simulink model "walkingRobotCapture"  (R2020a)
settings: Solver=ode15s  StartTime=0.0  StopTime=inf  EnableMultiTasking=on
PreLoadFcn:
  | % run script to load up the parameters
  | robotParameters
values from neighbouring files (symbols this model uses):
  foot_x = 0.17    [robotParameters.m]
  foot_y = 0.17    [robotParameters.m]
  foot_z = 0.02    [robotParameters.m]
  init_angs_L = zeros(6,1)    [robotParameters.m]
  init_angs_R = zeros(6,1)    [robotParameters.m]
  leg_width = 0.08    [robotParameters.m]
  lower_leg_length = 0.38    [robotParameters.m]
  plane_x = 3    [robotParameters.m]    (also in startupWalkingRobot.m = 30)
  plane_y = 50    [robotParameters.m]
  plane_z = height_plane    (= 0.025)    [robotParameters.m]
  s = Rp(:,2)    [invKinBody2Foot.m]
  torso_height = 0.35    [robotParameters.m]
  torso_length = 0.20    (= 0.2)    [robotParameters.m]
  torso_offset_height = 0    [robotParameters.m]
  torso_offset_length = 0    [robotParameters.m]
  torso_width = 0.24    [robotParameters.m]
  Ts = 0.005    [startupWalkingRobot.m]
  upper_leg_length = 0.40    (= 0.4)    [robotParameters.m]
  X = mat(1,4)    [Transform.m]
  Y = mat(2,4)    [Transform.m]
  Z = mat(3,4)    [Transform.m]
libraries: sm_lib x57, walkingRobotUtils x17, nesl_utility x4, simulink x1
(part 2 of 3)

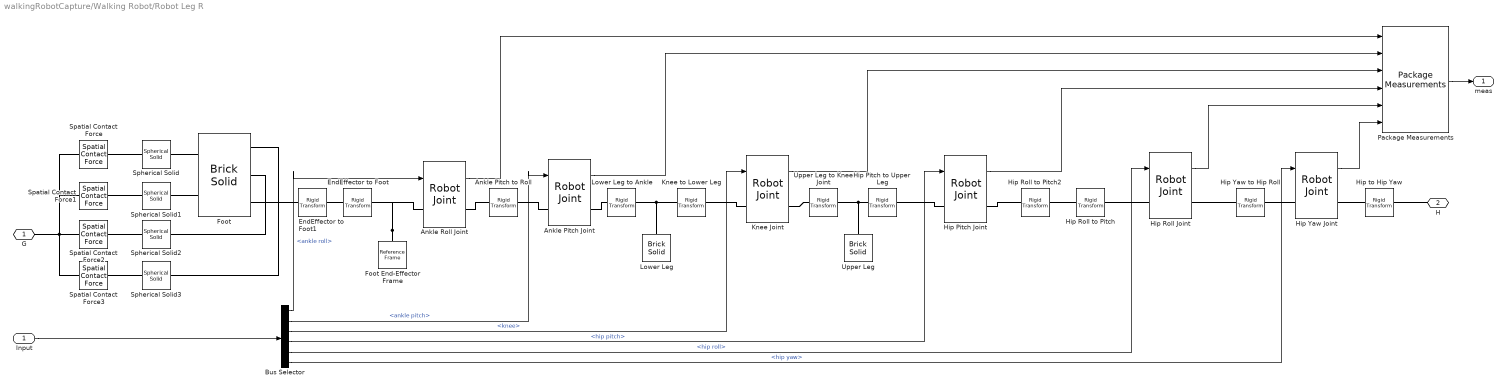
== system walkingRobotCapture/Walking Robot/Robot Leg R ==
  Input : Inport
  Ankle Pitch Joint : walkingRobotUtils/Robot Joint  jointDamping=joint_damping  initAngle=init_angs_R(5)  upperLimit=pi/2  lowerLimit=-pi/2  limitK=1000  limitD=100
  Ankle Pitch to Roll : sm_lib/Frames and Transforms/Rigid Transform  TranslationMethod=None  TranslationStandardOffset=0  TranslationLengthUnit=cm  TranslationStandardAxis=+Z  TranslationCartesianOffset=[0 0 upper_leg_length/2]  TranslationROffset=0  TranslationROffsetUnits=m  TranslationZOffset=0  TranslationZOffsetUnits=m  TranslationThetaOffset=0  TranslationThetaOffsetUnits=deg  RotationMethod=StandardAxis  RotationAngleUnits=deg  RotationStandardAxis=+X  RotationAngle=90  RotationArbitraryAxis=[0 0 1]  FollAlignAxisA=+X  BaseAlignAxisA=+Y  FollAlignAxisB=+Y  BaseAlignAxisB=+Z  RotationSequenceAxes=FollowerAxes  RotationSequence=XYX  RotationSequenceAngles=[0 0 0]  RotationSequenceAnglesUnits=deg  RotationMatrix=[1 0 0; 0 1 0; 0 0 1]
  Ankle Roll Joint : walkingRobotUtils/Robot Joint  jointDamping=joint_damping  initAngle=init_angs_R(6)  upperLimit=pi/2  lowerLimit=-pi/2  limitK=1000  limitD=100
  Bus Selector : BusSelector  OutputSignals=ankle roll,ankle pitch,knee,hip pitch,hip roll,hip yaw
  EndEffector to Foot : sm_lib/Frames and Transforms/Rigid Transform  TranslationMethod=None  TranslationStandardOffset=0  TranslationLengthUnit=cm  TranslationStandardAxis=+Z  TranslationCartesianOffset=[0 0 upper_leg_length/2]  TranslationROffset=0  TranslationROffsetUnits=m  TranslationZOffset=0  TranslationZOffsetUnits=m  TranslationThetaOffset=0  TranslationThetaOffsetUnits=deg  RotationMethod=StandardAxis  RotationAngleUnits=deg  RotationStandardAxis=+Z  RotationAngle=-90  RotationArbitraryAxis=[0 0 1]  FollAlignAxisA=+X  BaseAlignAxisA=+Y  FollAlignAxisB=+Y  BaseAlignAxisB=+Z  RotationSequenceAxes=FollowerAxes  RotationSequence=XYX  RotationSequenceAngles=[0 0 0]  RotationSequenceAnglesUnits=deg  RotationMatrix=[1 0 0; 0 1 0; 0 0 1]
  EndEffector to Foot1 : sm_lib/Frames and Transforms/Rigid Transform  TranslationMethod=None  TranslationStandardOffset=0  TranslationLengthUnit=cm  TranslationStandardAxis=+Z  TranslationCartesianOffset=[0 0 upper_leg_length/2]  TranslationROffset=0  TranslationROffsetUnits=m  TranslationZOffset=0  TranslationZOffsetUnits=m  TranslationThetaOffset=0  TranslationThetaOffsetUnits=deg  RotationMethod=StandardAxis  RotationAngleUnits=deg  RotationStandardAxis=+X  RotationAngle=180  RotationArbitraryAxis=[0 0 1]  FollAlignAxisA=+X  BaseAlignAxisA=+Y  FollAlignAxisB=+Y  BaseAlignAxisB=+Z  RotationSequenceAxes=FollowerAxes  RotationSequence=XYX  RotationSequenceAngles=[0 0 0]  RotationSequenceAnglesUnits=deg  RotationMatrix=[1 0 0; 0 1 0; 0 0 1]
  Foot : sm_lib/Body Elements/Brick Solid  GraphicAmbientColor=[0.15 0.15 0.15 1.0]  BasedOnType=Density  BrickDimensions=[foot_x foot_y foot_z]  BrickDimensionUnits=m  CenterOfMass=[0 0 0]  CenterOfMassUnits=m  GraphicDiffuseColor=[0.5 0.5 0.5]  Density=200  DensityUnits=kg/(m^3)  DoExposeReferenceFrame=off  GraphicEmissiveColor=[0.0 0.0 0.0 1.0]  ExportEntireGeometry=off  SerializedFrames=<Frames><Frame><Id>Frame1</Id><Value><Name>F1</Name><Origin><Source>GeometricFeature</Source><FeatureName>+x -y curve</FeatureName></Origin><PrimaryAxis><DefinedDirection>+Z</DefinedDirection><Source>ReferenceFrame</Source><SourceDirection>+Z</SourceDirection><FeatureName></FeatureName></PrimaryAxis><SecondaryAxis><DefinedDirection>+X</DefinedDirection><Source>ReferenceFrame</Source><SourceDirection>+X</SourceDirection><FeatureName></FeatureName></SecondaryAxis></Value></Frame><Frame><Id>Frame2</Id><Value><Name>F2</Name><Origin><Source>GeometricFeature</Source><FeatureName>+x +y curve</FeatureName></Origin><PrimaryAxis><DefinedDirection>+Z</DefinedDirection><Source>ReferenceFrame</Source><SourceDirection>+Z</SourceDirection><FeatureName></FeatureName></PrimaryAxis><SecondaryAxis><DefinedDirection>+X</DefinedDirection><Source>ReferenceFrame</Source><SourceDirection>+X</SourceDirection><FeatureName></FeatureName></SecondaryAxis></Value></Frame><Frame><Id>Frame3</Id><Value><Name>F3</Name><Origin><Source>GeometricFeature</Source><FeatureName>-x -y curve</FeatureName></Origin><PrimaryAxis><DefinedDirection>+Z</DefinedDirection><Source>ReferenceFrame</Source><SourceDirection>+Z</SourceDirection><FeatureName></FeatureName></PrimaryAxis><SecondaryAxis><DefinedDirection>+X</DefinedDirection><Source>ReferenceFrame</Source><SourceDirection>+X</SourceDirection><FeatureName></FeatureName></SecondaryAxis></Value></Frame><Frame><Id>Frame4</Id><Value><Name>F4</Name><Origin><Source>GeometricFeature</Source><FeatureName>-x +y curve</FeatureName></Origin><PrimaryAxis><DefinedDirection>+Z</DefinedDirection><Source>ReferenceFrame</Source><SourceDirection>+Z</SourceDirection><FeatureName></FeatureName></PrimaryAxis><SecondaryAxis><DefinedDirection>+X</DefinedDirection><Source>ReferenceFrame</Source><SourceDirection>+X</SourceDirection><FeatureName></FeatureName></SecondaryAxis></Value></Frame><Frame><Id>Frame5</Id><Value><Name>A</Name><Origin><Source>GeometricFeature</Source><FeatureName>+z surface</FeatureName></Origin><PrimaryAxis><DefinedDirection>+Z</DefinedDirection><Source>ReferenceFrame</Source><SourceDirection>-Y</SourceDirection><FeatureName></FeatureName></PrimaryAxis><SecondaryAxis><DefinedDirection>+X</DefinedDirection><Source>ReferenceFrame</Source><SourceDirection>+X</SourceDirection><FeatureName></FeatureName></SecondaryAxis></Value></Frame></Frames>  MarkerShape=Sphere  MarkerSize=10  GraphicType=FromGeometry  InertiaType=CalculateFromGeometry  Mass=1  MassUnits=kg  MomentsOfInertia=[1 1 1]  MomentsOfInertiaUnits=kg*m^2  GraphicOpacity=1.0  ProductsOfInertia=[0 0 0]  ProductsOfInertiaUnits=kg*m^2  GraphicShininess=75  GraphicSpecularColor=[0.5 0.5 0.5 1.0]  GraphicVisPropType=SimpleVisualProperties
  Foot End-Effector Frame : sm_lib/Frames and Transforms/Reference Frame
  Hip Pitch Joint : walkingRobotUtils/Robot Joint  jointDamping=joint_damping  initAngle=init_angs_R(3)  upperLimit=pi/2  lowerLimit=-pi/2  limitK=1000  limitD=100
  Hip Pitch to Upper Leg : sm_lib/Frames and Transforms/Rigid Transform  TranslationMethod=StandardAxis  TranslationStandardOffset=upper_leg_length/2  TranslationLengthUnit=m  TranslationStandardAxis=+X  TranslationCartesianOffset=[upper_leg_length/2 0 0]  TranslationROffset=0  TranslationROffsetUnits=m  TranslationZOffset=0  TranslationZOffsetUnits=m  TranslationThetaOffset=0  TranslationThetaOffsetUnits=deg  RotationMethod=StandardAxis  RotationAngleUnits=deg  RotationStandardAxis=+Y  RotationAngle=90  RotationArbitraryAxis=[0 0 1]  FollAlignAxisA=+X  BaseAlignAxisA=+Y  FollAlignAxisB=+Y  BaseAlignAxisB=+Z  RotationSequenceAxes=FollowerAxes  RotationSequence=XYX  RotationSequenceAngles=[0 0 0]  RotationSequenceAnglesUnits=deg  RotationMatrix=[1 0 0; 0 1 0; 0 0 1]
  Hip Roll Joint : walkingRobotUtils/Robot Joint  jointDamping=joint_damping  initAngle=init_angs_R(2)  upperLimit=pi/2  lowerLimit=-pi/2  limitK=1000  limitD=100
  Hip Roll to Pitch : sm_lib/Frames and Transforms/Rigid Transform  TranslationMethod=None  TranslationStandardOffset=0  TranslationLengthUnit=cm  TranslationStandardAxis=+Z  TranslationCartesianOffset=[0 0 upper_leg_length/2]  TranslationROffset=0  TranslationROffsetUnits=m  TranslationZOffset=0  TranslationZOffsetUnits=m  TranslationThetaOffset=0  TranslationThetaOffsetUnits=deg  RotationMethod=StandardAxis  RotationAngleUnits=deg  RotationStandardAxis=+Z  RotationAngle=-90  RotationArbitraryAxis=[0 0 1]  FollAlignAxisA=+X  BaseAlignAxisA=+Y  FollAlignAxisB=+Y  BaseAlignAxisB=+Z  RotationSequenceAxes=FollowerAxes  RotationSequence=XYX  RotationSequenceAngles=[0 0 0]  RotationSequenceAnglesUnits=deg  RotationMatrix=[1 0 0; 0 1 0; 0 0 1]
  Hip Roll to Pitch2 : sm_lib/Frames and Transforms/Rigid Transform  TranslationMethod=None  TranslationStandardOffset=0  TranslationLengthUnit=cm  TranslationStandardAxis=+Z  TranslationCartesianOffset=[0 0 upper_leg_length/2]  TranslationROffset=0  TranslationROffsetUnits=m  TranslationZOffset=0  TranslationZOffsetUnits=m  TranslationThetaOffset=0  TranslationThetaOffsetUnits=deg  RotationMethod=StandardAxis  RotationAngleUnits=deg  RotationStandardAxis=+X  RotationAngle=-90  RotationArbitraryAxis=[0 0 1]  FollAlignAxisA=+X  BaseAlignAxisA=+Y  FollAlignAxisB=+Y  BaseAlignAxisB=+Z  RotationSequenceAxes=FollowerAxes  RotationSequence=XYX  RotationSequenceAngles=[0 0 0]  RotationSequenceAnglesUnits=deg  RotationMatrix=[1 0 0; 0 1 0; 0 0 1]
  Hip Yaw Joint : walkingRobotUtils/Robot Joint  jointDamping=joint_damping  initAngle=init_angs_R(1)  upperLimit=pi/2  lowerLimit=-pi/2  limitK=1000  limitD=100
  Hip Yaw to Hip Roll : sm_lib/Frames and Transforms/Rigid Transform  TranslationMethod=None  TranslationStandardOffset=0  TranslationLengthUnit=cm  TranslationStandardAxis=+Z  TranslationCartesianOffset=[0 0 upper_leg_length/2]  TranslationROffset=0  TranslationROffsetUnits=m  TranslationZOffset=0  TranslationZOffsetUnits=m  TranslationThetaOffset=0  TranslationThetaOffsetUnits=deg  RotationMethod=StandardAxis  RotationAngleUnits=deg  RotationStandardAxis=+X  RotationAngle=90  RotationArbitraryAxis=[0 0 1]  FollAlignAxisA=+X  BaseAlignAxisA=+Y  FollAlignAxisB=+Y  BaseAlignAxisB=+Z  RotationSequenceAxes=FollowerAxes  RotationSequence=XYX  RotationSequenceAngles=[0 0 0]  RotationSequenceAnglesUnits=deg  RotationMatrix=[1 0 0; 0 1 0; 0 0 1]
  Hip to Hip Yaw : sm_lib/Frames and Transforms/Rigid Transform  TranslationMethod=None  TranslationStandardOffset=0  TranslationLengthUnit=cm  TranslationStandardAxis=+Z  TranslationCartesianOffset=[0 0 upper_leg_length/2]  TranslationROffset=0  TranslationROffsetUnits=m  TranslationZOffset=0  TranslationZOffsetUnits=m  TranslationThetaOffset=0  TranslationThetaOffsetUnits=deg  RotationMethod=StandardAxis  RotationAngleUnits=deg  RotationStandardAxis=+Z  RotationAngle=180  RotationArbitraryAxis=[0 0 1]  FollAlignAxisA=+X  BaseAlignAxisA=+Y  FollAlignAxisB=+Y  BaseAlignAxisB=+Z  RotationSequenceAxes=FollowerAxes  RotationSequence=XYX  RotationSequenceAngles=[0 0 0]  RotationSequenceAnglesUnits=deg  RotationMatrix=[1 0 0; 0 1 0; 0 0 1]
  Knee Joint : walkingRobotUtils/Robot Joint  jointDamping=joint_damping  initAngle=init_angs_R(4)  upperLimit=pi/2  lowerLimit=-pi/2  limitK=1000  limitD=100
  Knee to Lower Leg : sm_lib/Frames and Transforms/Rigid Transform  TranslationMethod=StandardAxis  TranslationStandardOffset=lower_leg_length/2  TranslationLengthUnit=m  TranslationStandardAxis=+X  TranslationCartesianOffset=[upper_leg_length/2 0 0]  TranslationROffset=0  TranslationROffsetUnits=m  TranslationZOffset=0  TranslationZOffsetUnits=m  TranslationThetaOffset=0  TranslationThetaOffsetUnits=deg  RotationMethod=StandardAxis  RotationAngleUnits=deg  RotationStandardAxis=+Y  RotationAngle=90  RotationArbitraryAxis=[0 0 1]  FollAlignAxisA=+X  BaseAlignAxisA=+Y  FollAlignAxisB=+Y  BaseAlignAxisB=+Z  RotationSequenceAxes=FollowerAxes  RotationSequence=XYX  RotationSequenceAngles=[0 0 0]  RotationSequenceAnglesUnits=deg  RotationMatrix=[1 0 0; 0 1 0; 0 0 1]
  Lower Leg : sm_lib/Body Elements/Brick Solid  GraphicAmbientColor=[0.15 0.15 0.15 1.0]  BasedOnType=Density  BrickDimensions=[leg_width leg_width lower_leg_length]  BrickDimensionUnits=m  CenterOfMass=[0 0 0]  CenterOfMassUnits=m  GraphicDiffuseColor=[0.4 0.4 1.0]  Density=200  DensityUnits=kg/m^3  DoExposeReferenceFrame=on  GraphicEmissiveColor=[0.0 0.0 0.0 1.0]  ExportEntireGeometry=off  SerializedFrames=<Frames/>  MarkerShape=Sphere  MarkerSize=10  GraphicType=FromGeometry  InertiaType=CalculateFromGeometry  Mass=1  MassUnits=kg  MomentsOfInertia=[1 1 1]  MomentsOfInertiaUnits=kg*m^2  GraphicOpacity=1.0  ProductsOfInertia=[1 1 1]  ProductsOfInertiaUnits=kg*m^2  GraphicShininess=75  GraphicSpecularColor=[0.5 0.5 0.5 1.0]  GraphicVisPropType=SimpleVisualProperties
  Lower Leg to Ankle : sm_lib/Frames and Transforms/Rigid Transform  TranslationMethod=StandardAxis  TranslationStandardOffset=lower_leg_length/2  TranslationLengthUnit=m  TranslationStandardAxis=+Z  TranslationCartesianOffset=[upper_leg_length/2 0 0]  TranslationROffset=0  TranslationROffsetUnits=m  TranslationZOffset=0  TranslationZOffsetUnits=m  TranslationThetaOffset=0  TranslationThetaOffsetUnits=deg  RotationMethod=StandardAxis  RotationAngleUnits=deg  RotationStandardAxis=+Y  RotationAngle=-90  RotationArbitraryAxis=[0 0 1]  FollAlignAxisA=+X  BaseAlignAxisA=+Y  FollAlignAxisB=+Y  BaseAlignAxisB=+Z  RotationSequenceAxes=FollowerAxes  RotationSequence=XYX  RotationSequenceAngles=[0 0 0]  RotationSequenceAnglesUnits=deg  RotationMatrix=[1 0 0; 0 1 0; 0 0 1]
  Package Measurements : walkingRobotUtils/Package Measurements  SystemSampleTime=-1  Latency=0  AutoFrameSizeCalculation=off
  Spatial Contact Force{,1..3} (4 alike) : sm_lib/Forces and Torques/Spatial Contact Force  CoefficientOfDynamicFriction=mu_k  CoefficientOfStaticFriction=mu_s  NormalDamping=contact_damping  NormalDampingUnits=N/(m/s)  NormalStiffness=contact_stiffness  NormalStiffnessUnits=N/m  FrictionalCriticalVelocity=mu_vth  FrictionalCriticalVelocityUnits=m/s  ZeroCrossDetectContactStartAndEnd=off  SenseFrictionalForceMagnitude=off  SenseNormalForceMagnitude=off  SenseSeparationDistance=off  NormalTransitionRegionWidth=1e-4  NormalTransitionRegionWidthUnits=m  FrictionType=SmoothStickSlip
  Spherical Solid{,1..3} (4 alike) : sm_lib/Body Elements/Spherical Solid  GraphicAmbientColor=[0.15 0.15 0.15 1.0]  BasedOnType=Mass  CenterOfMass=[0 0 0]  CenterOfMassUnits=m  GraphicDiffuseColor=[0.5 0.5 0.5]  Density=1000  DensityUnits=kg/m^3  DoExposeReferenceFrame=on  GraphicEmissiveColor=[0.0 0.0 0.0 1.0]  ExportEntireGeometry=on  SerializedExposedGeometries=<ExposedGeometries><ExposedGeometry><RawGeometryId>entire</RawGeometryId><ExposedGeometryId>G</ExposedGeometryId></ExposedGeometry></ExposedGeometries>  SerializedFrames=<Frames/>  MarkerShape=Sphere  MarkerSize=10  GraphicType=FromGeometry  InertiaType=CalculateFromGeometry  Mass=1  MassUnits=g  MomentsOfInertia=[1 1 1]  MomentsOfInertiaUnits=kg*m^2  GraphicOpacity=1.0  ProductsOfInertia=[0 0 0]  ProductsOfInertiaUnits=kg*m^2  GraphicShininess=75  GraphicSpecularColor=[0.5 0.5 0.5 1.0]  SphereRadius=foot_z/2  SphereRadiusUnits=m  GraphicVisPropType=SimpleVisualProperties
  Upper Leg : sm_lib/Body Elements/Brick Solid  GraphicAmbientColor=[0.15 0.15 0.15 1.0]  BasedOnType=Density  BrickDimensions=[leg_width leg_width upper_leg_length]  BrickDimensionUnits=m  CenterOfMass=[0 0 0]  CenterOfMassUnits=m  GraphicDiffuseColor=[1.0 0.4 0.4]  Density=200  DensityUnits=kg/m^3  DoExposeReferenceFrame=on  GraphicEmissiveColor=[0.0 0.0 0.0 1.0]  ExportEntireGeometry=off  SerializedFrames=<Frames/>  MarkerShape=Sphere  MarkerSize=10  GraphicType=FromGeometry  InertiaType=CalculateFromGeometry  Mass=1  MassUnits=kg  MomentsOfInertia=[1 1 1]  MomentsOfInertiaUnits=kg*m^2  GraphicOpacity=1.0  ProductsOfInertia=[1 1 1]  ProductsOfInertiaUnits=kg*m^2  GraphicShininess=75  GraphicSpecularColor=[0.5 0.5 0.5 1.0]  GraphicVisPropType=SimpleVisualProperties
  Upper Leg to Knee Joint : sm_lib/Frames and Transforms/Rigid Transform  TranslationMethod=StandardAxis  TranslationStandardOffset=upper_leg_length/2  TranslationLengthUnit=m  TranslationStandardAxis=+Z  TranslationCartesianOffset=[upper_leg_length/2 0 0]  TranslationROffset=0  TranslationROffsetUnits=m  TranslationZOffset=0  TranslationZOffsetUnits=m  TranslationThetaOffset=0  TranslationThetaOffsetUnits=deg  RotationMethod=StandardAxis  RotationAngleUnits=deg  RotationStandardAxis=+Y  RotationAngle=-90  RotationArbitraryAxis=[0 0 1]  FollAlignAxisA=+X  BaseAlignAxisA=+Y  FollAlignAxisB=+Y  BaseAlignAxisB=+Z  RotationSequenceAxes=FollowerAxes  RotationSequence=XYX  RotationSequenceAngles=[0 0 0]  RotationSequenceAnglesUnits=deg  RotationMatrix=[1 0 0; 0 1 0; 0 0 1]
  G : PMIOPort  Side=Right
  H : PMIOPort  Port=2  Side=Right
  meas : Outport  VectorParamsAs1DForOutWhenUnconnected=off
  wires:
  Ankle Roll Joint/1 -> Package Measurements/1
  Bus Selector/1 -> Ankle Roll Joint/1  "<ankle roll>"
  Hip Yaw Joint/1 -> Package Measurements/6
  Hip Roll Joint/1 -> Package Measurements/5
  Bus Selector/6 -> Hip Yaw Joint/1  "<hip yaw>"
  Bus Selector/5 -> Hip Roll Joint/1  "<hip roll>"
  Bus Selector/2 -> Ankle Pitch Joint/1  "<ankle pitch>"
  Bus Selector/3 -> Knee Joint/1  "<knee>"
  Bus Selector/4 -> Hip Pitch Joint/1  "<hip pitch>"
  Package Measurements/1 -> meas/1
  Hip Pitch Joint/1 -> Package Measurements/4
  Knee Joint/1 -> Package Measurements/3
  Ankle Pitch Joint/1 -> Package Measurements/2
  Input/1 -> Bus Selector/1
  connections:
  Spatial Contact Force2/RConn1 -- Spherical Solid2/LConn1
  Spherical Solid/LConn1 -- Spatial Contact Force/RConn1
  Spherical Solid1/RConn1 -- Foot/RConn2
  Spherical Solid2/RConn1 -- Foot/LConn2
  Spherical Solid1/LConn1 -- Spatial Contact Force1/RConn1
  Spherical Solid3/LConn1 -- Spatial Contact Force3/RConn1
  Spherical Solid3/RConn1 -- Foot/LConn1
  EndEffector to Foot1/RConn1 -- Foot/LConn3
  Spherical Solid/RConn1 -- Foot/RConn1
  Spatial Contact Force3/LConn1 -- G/RConn1 -- Spatial Contact Force1/LConn1 -- Spatial Contact Force/LConn1 -- Spatial Contact Force2/LConn1
  Upper Leg to Knee Joint/LConn1 -- Hip Pitch to Upper Leg/RConn1 -- Upper Leg/RConn1
  Lower Leg to Ankle/LConn1 -- Knee to Lower Leg/RConn1 -- Lower Leg/RConn1
  Ankle Roll Joint/RConn1 -- Ankle Pitch to Roll/RConn1
  Foot End-Effector Frame/RConn1 -- Ankle Roll Joint/LConn1 -- EndEffector to Foot/LConn1
  EndEffector to Foot1/LConn1 -- EndEffector to Foot/RConn1
  Ankle Pitch Joint/LConn1 -- Ankle Pitch to Roll/LConn1
  Hip Pitch Joint/LConn1 -- Hip Pitch to Upper Leg/LConn1
  Hip Yaw Joint/RConn1 -- Hip to Hip Yaw/RConn1
  Hip Roll to Pitch2/LConn1 -- Hip Roll to Pitch/RConn1
  Hip Roll Joint/LConn1 -- Hip Roll to Pitch/LConn1
  Hip Roll Joint/RConn1 -- Hip Yaw to Hip Roll/RConn1
  Hip Yaw Joint/LConn1 -- Hip Yaw to Hip Roll/LConn1
  Hip Pitch Joint/RConn1 -- Hip Roll to Pitch2/RConn1
  Hip to Hip Yaw/LConn1 -- H/RConn1
  Knee Joint/RConn1 -- Upper Leg to Knee Joint/RConn1
  Ankle Pitch Joint/RConn1 -- Lower Leg to Ankle/RConn1
  Knee Joint/LConn1 -- Knee to Lower Leg/LConn1

== matlab function walkingRobotCapture/Inverse Kinematics/Inverse Kinematics L ==
  data: transmat input; q output; isLeft input
function q = inverseKinematics(transmat, isLeft)
q = invKinBody2Foot(transmat, isLeft);

== matlab function walkingRobotCapture/Inverse Kinematics/Inverse Kinematics R ==
  data: transmat input; q output; isLeft input
function q = inverseKinematics(transmat, isLeft)
q = invKinBody2Foot(transmat, isLeft);

== stateflow chart walkingRobotCapture/Trajectory Planner ==
  state StandBy
    entry:
    idxmax = 0.5/TS;
    during:
    idx = idx + 1;
  note: eos: End of step
      | Tb_bp: body prime (body at eos) to body
      | Tw_b: body to world
      | Tw_f: transform from world to foot
      | Capture point-end-of-step (cp-eos) is where you want the capture point
      | to be at the end of the step.
      | cxeos: capture point (x) end of step
      | cyeos: capture point (y) end of step
      | And remember, in this example, foot position is set to be positioned at
      | the cp-eos. In the paper, Englesberger set it with some offset.
  state BendKnee
    entry:
    endPoseRight =           [0 -1 0 0.12;0 0 1 0;-1 0 0 -0.78;0 0 0 1];
    endPoseRightTarget = [0 -1 0 0.12;0 0 1 0;-1 0 0 -ZMODEL;0 0 0 1];
    endPoseLeft =          [0 -1 0 -0.12;0 0 1 0;-1 0 0 -0.78;0 0 0 1];
    endPoseLeftTarget =[0 -1 0 -0.12;0 0 1 0;-1 0 0 -ZMODEL;0 0 0 1];
    tduration = 1.5;
    xyzqtrajr = generateTraj(endPoseRight, endPoseRightTarget, tduration);
    xyzqtrajl = generateTraj(endPoseLeft, endPoseLeftTarget, tduration);
    idx = 1; idxmax = round(tduration/TS);
    endPoseRight = xyzq2Tform(xyzqtrajr(:,idx));
    endPoseLeft = xyzq2Tform(xyzqtrajl(:,idx));
    idx = idx + 1;
    during:
    endPoseRight = xyzq2Tform(xyzqtrajr(:,idx));
    endPoseLeft = xyzq2Tform(xyzqtrajl(:,idx));
    idx = idx + 1;
  state RightStance
    entry:
    calculateRightTrajectories();
    during:
    %endPoseRight(1:3,4) = xyzqtrajr(1:3,idx); %stancetraj(:,idx);
    %endPoseLeft(1:3,4) = xyzqtrajl(1:3,idx);
    endPoseRight = xyzq2Tform(xyzqtrajr(:,idx));
    endPoseLeft = xyzq2Tform(xyzqtrajl(:,idx));
    idx = idx + 1;
  state LeftStance
    entry:
    calculateLeftTrajectories();
    during:
    %endPoseLeft(1:3,4) = stancetraj(:,idx);
    %endPoseRight(1:3,4) = xyzqtrajr(1:3,idx);
    endPoseLeft = xyzq2Tform(xyzqtrajl(:,idx));
    endPoseRight = xyzq2Tform(xyzqtrajr(:,idx));
    idx = idx + 1;
  state WalkReady
    entry:
    endPoseRight = endPoseRightTarget;
    endPoseLeft = endPoseLeftTarget;
    endPoseRightTarget(1:3,4) = [0.0; 0.0; -ZMODEL];
    endPoseLeftTarget(1:3,4) = [-0.24; 0.0; -ZMODEL];
    tduration = 1.5;
    xyzqtrajr = generateTraj(endPoseRight, endPoseRightTarget, tduration);
    xyzqtrajl = generateTraj(endPoseLeft, endPoseLeftTarget, tduration);
    idxmax = round(tduration/TS);
    endPoseRight = xyzq2Tform(xyzqtrajr(:,idx));
    endPoseLeft = xyzq2Tform(xyzqtrajl(:,idx));
    idx = idx + 1;
    during:
    endPoseRight = xyzq2Tform(xyzqtrajr(:,idx));
    endPoseLeft = xyzq2Tform(xyzqtrajl(:,idx));
    idx = idx + 1;
  (default) -> StandBy : {idx = 1;}
  StandBy -> BendKnee : [idx > idxmax]
      | {idx = 1;}
  RightStance -> LeftStance : [idx > idxmax]{idx = 1;}
  LeftStance -> RightStance : [idx > idxmax]{idx = 1;}
  BendKnee -> WalkReady : [idx > idxmax]
      | {idx = 1;}
  WalkReady -> RightStance : [idx > idxmax]
      | {idx = 1;}
  data: xyzq function_input; tform function_output; currMat function_input; targetMat function_input; taction function_input; xyzqtrajectory function_output; initialstate function_input; initialinput function_input; measurementvec function_output; statef function_output; maxidx function_input; cpointx function_input; cpointy function_input; w function_input; dT function_input; pX function_output; pY function_output; cpdesiredx function_input; cpdesiredy function_input; currMat function_input; targetMat function_input; xyzqtrajectory function_output; liptraj function_input; cpointx function_input; cpointy function_input; straj function_output; state_ function_input; w_ function_input; capturepointx function_output; capturepointy function_output; currMat function_input; targetMat function_input; xyzqtrajectory function_output; liptraj function_input; cpointx function_input; cpointy function_input; currMat function_input; targetMat function_input; tformtrajectory function_output; currMat function_input; targetMat function_input; xyzqtrajectory function_output; Tw_b_traj function_input; Tw_f_mat function_input; endPoseRight output =[0 -1 0 0.12;0 0 1 0;-1 0 0 -0.78;0 0 0 1]; endPoseLeft output =[0 -1 0 -0.12;0 0 1 0;-1 0 0 -0.78;0 0 0 1]; TS constant double =Ts; idx local; idxmax local size=1; BD constant double size=[4 2] =Bd; AD constant double size=[4 4] =Ad; CD constant double size=[2 4] =Cd; DD constant double size=[2 2] =Dd; STEPTIME constant double =desiredStepTime; state0 local =[x0 dx0 y0 dy0]'; u0 local =[px0 py0]'; meas1 local; state1 local size=[4,1] =zeros(4,1); measvec local =zeros(3,250); temp local; W constant double =w; py local; px local; ZMODEL constant double =zModel; stancetraj local; cy local; cx local; endPoseRightTarget local; endPoseLeftTarget local; xyzqtrajr local size=[7, 2500]; xyzqtrajl local size=[7, 2500]; tduration local; Tw_b local =eye(4); fholdy local; fholdx local; cxeos local; deltaPos input; cyeos local; SWINGHEIGHT constant double =0.1; deltaYaw input; Tb_bp local =eye(4); Tw_f local =zeros(4); TB_FL constant double size=[4,4] =[0 -1 0 -0.12;0 0 1 0;-1 0 0 -zModel;0 0 0 1];; TB_FR constant double size=[4,4] =[0 -1 0 0.12;0 0 1 0;-1 0 0 -zModel;0 0 0 1];; Tb_fl local size=[4,4]; Tb_fr local size=[4,4]; tformtrajl local size=[4,4,1000]; tformtrajr local size=[4,4,1000]
  function tform = xyzq2Tform(xyzq):
    | function tform = xyzq2Tform(xyzq)
    | 
    | val = reshape(xyzq(4:7),1,4); 
    | q = quaternion(val); 
    | rmat = q.rotmat('frame');
    | tform = eye(4);
    | tform(1:3,1:3) = rmat; 
    | tform(1:3,4) = xyzq(1:3);
  function xyzqtrajectory = generateTraj(currMat, targetMat, taction):
    | function xyzqtrajectory = generateTraj(currMat, targetMat, taction)
    | 
    | quat = quaternion(currMat(1:3,1:3), 'rotmat', 'frame'); 
    | quat = quat.compact; 
    | quattarget = quaternion(targetMat(1:3,1:3), 'rotmat', 'frame');
    | quattarget = quattarget.compact; 
    | 
    | x = currMat(1,4); y = currMat(2,4); z = currMat(3,4); 
    | xt = targetMat(1,4); yt = targetMat(2,4); zt = targetMat(3,4); 
    | 
    | currPts = [x y z quat]';
    | targetPts = [xt yt zt quattarget]'; 
    | 
    | wpts = [currPts targetPts]; 
    | tpts = [0 taction];
    | tvec = 0:TS:taction; 
    | 
    | [xyzqtrajectory, ~, ~, ~] = cubicpolytraj(wpts, tpts, tvec);
  function [measurementvec, statef] = simulateLipm(initialstate, initialinput, maxidx):
    | function [measurementvec, statef] = simulateLipm(initialstate, initialinput, maxidx)
    |     state0 = initialstate; 
    |     u0 = initialinput; 
    |     measurementvec = zeros(3,250); 
    |     measurementvec(3,:) = ZMODEL; 
    |     
    |     meas1 = CD*state0 + DD*u0;
    |     measurementvec(1:2,1) = meas1;
    |     for temp = 2:maxidx
    |         state1 = AD*state0 + BD*u0;
    |         meas1  = CD*state1 + DD*u0;
    |         measurementvec(1:2,temp) = meas1;
    |         state0 = state1;
    |     end
    |     statef = state1; 
    | end 
    | % meas1 = CD*state0 + DD*u0;
    | % measvec(1:2,1) = meas1;
    | % for temp = 2:idxmax
    | %     state1 = AD*state0 + BD*u0;
    | %     meas1  = CD*state1 + DD*u0;
    | %     measvec(1:2,temp) = meas1;
    | %     state0 = state1;
    | % end
  function [pX,pY] = findZmp(cpointx, cpointy, w, dT, cpdesiredx, cpdesiredy):
    | function [pX,pY] = findZmp(cpointx, cpointy, w, dT, cpdesiredx, cpdesiredy)
    | b = exp(w*dT); 
    | pX = 1/(1-b)*cpdesiredx - b/(1-b)*cpointx; 
    | pY = 1/(1-b)*cpdesiredy - b/(1-b)*cpointy; 
    | end
  function xyzqtrajectory = generateSwingTraj(currMat, targetMat):
    | function xyzqtrajectory = generateSwingTraj(currMat, targetMat)
    | 
    | quat = quaternion(currMat(1:3,1:3), 'rotmat', 'frame'); 
    | quat = quat.compact; 
    | quattarget = quaternion(targetMat(1:3,1:3), 'rotmat', 'frame');
    | quattarget = quattarget.compact; 
    | 
    | x0 = currMat(1,4);     y0 = currMat(2,4);     z0 = currMat(3,4); 
    | x2 = targetMat(1,4);   y2 = targetMat(2,4);   z2 = targetMat(3,4); 
    | x1 = (x0 + x2)/2;      y1 = (y0 + y2)/2;      z1 = z0 + SWINGHEIGHT; 
    | 
    | pts0 = [x0 y0 z0 quat]';
    | pts1 = [x1 y1 z1 quattarget]'; 
    | pts2 = [x2 y2 z2 quattarget]'; 
    | 
    | wpts = [pts0 pts1 pts2]; 
    | tpts = [0 STEPTIME/2 STEPTIME];
    | tvec = 0:TS:STEPTIME; 
    | 
    | [xyzqtrajectory, ~, ~, ~] = cubicpolytraj(wpts, tpts, tvec); 
    | end
  function straj = getStanceTraj(liptraj,cpointx, cpointy):
    | function straj = getStanceTraj(liptraj,cpointx, cpointy)
    | % transform body trajectory (w.r.t. world) to 
    | % foot trajectory (w.r.t. body) 
    | straj = -liptraj;
    | straj(1,:) = straj(1,:) + cpointx; 
    | straj(2,:) = straj(2,:) + cpointy; 
    | straj(3,:) = -ZMODEL; 
    | end
  function [capturepointx, capturepointy] = getCapturePoint(state_, w_):
    | function [capturepointx, capturepointy] = getCapturePoint(state_, w_)
    | xc = state_(1); 
    | yc = state_(3);
    | dxc = state_(2); 
    | dyc = state_(4); 
    | capturepointx = xc + dxc/w_; 
    | capturepointy = yc + dyc/w_; 
    | end
  function calculateRightTrajectories:
    | function calculateRightTrajectories
    | % transform from current body pose to next end of step body pose
    | Tb_bp = eye(4); 
    | Tb_bp(1,1) =  cos(deltaYaw); Tb_bp(1,2) = sin(deltaYaw);
    | Tb_bp(2,1) = -sin(deltaYaw); Tb_bp(2,2) = cos(deltaYaw);
    | Tb_bp(1,4) = deltaPos(1); 
    | Tb_bp(2,4) = deltaPos(2); 
    | 
    | % Tw_b: transform from world to body pose at end of step 
    | % Tw_f: transform from world to foot 
    | % Tb_fl: ''       from body to foot left
    | Tw_fr0 = Tw_b * TB_FR; % currrent world to right foot transform 
    | Tw_b   = Tw_b * Tb_bp; % next step world to body 
    | Tw_fr1 = Tw_b * TB_FR; % next world to right foot transform 
    | Tw_fl  = Tw_b * TB_FL;
    | % Tb_fl = Tb_bp * TB_FL; 
    | Tb_fr1 = Tb_bp * TB_FR; % end of step body to right foot transform 
    | cxeos  = Tw_fl(1,4);
    | cyeos  = Tw_fl(2,4);
    | 
    | % based on current capture point cx, cy and desired capture point at the
    | % end of step cxeos, cyeos, calculate the needed stance foot location (ZMP)
    | % px and py. 
    | [cx, cy] = getCapturePoint(state0,W);
    | [px, py] = findZmp(cx, cy, W, STEPTIME, cxeos, cyeos);
    | u0 = [px py]';
    | fholdx = cx;
    | fholdy = cy;
    | Tw_fr1(1,4) = fholdx; Tw_fr1(2,4) = fholdy; 
    | 
    | % the LIPM trajectory based on px, py (u0) will get you to where you want
    | % at the end of step 
    | idxmax = round(STEPTIME/TS);
    | [measvec, state1] = simulateLipm(state0, u0, idxmax);
    | state0 = state1;
    | % get world to new body pose based on state
    | Tw_bp = Tw_b;
    | Tw_bp(1,4) = state1(1); Tw_bp(2,4) = state1(3); 
    | % Get inverse
    | Tbp_w = eye(4);
    | Tbp_w(1:3,1:3) = Tw_bp(1:3,1:3)'; 
    | Tbp_w(1:3,4) = -Tw_bp(1:3,1:3)'*Tw_bp(1:3,4); 
    | Tbp_fl = Tbp_w * Tw_fl; 
    | 
    | % now translate those points into what robot can understand. Get the points
    | % w.r.t. the robot 
    | endPoseLeftTarget(1:3,1:3) = TB_FL(1:3,1:3); 
    | Tw_b(1,4) = state1(1); Tw_b(2,4) = state1(3); 
    | Tb_w = TransformInverse(Tw_b); 
    | Tb_fl = Tb_w * Tw_fl; 
    | endPoseLeftTarget(1,4) = Tb_fl(1,4); %cxeos - state1(1);
    | endPoseLeftTarget(2,4) = Tb_fl(2,4); %cyeos - state1(3);
    | % tformtrajl = generateSwingTraj2(endPoseLeft, endPoseLeftTarget); 
    | xyzqtrajl = generateSwingTraj(endPoseLeft, endPoseLeftTarget);
    | % stancetraj = getStanceTraj(measvec,fholdx,fholdy);
    | 
    | % only orientation will be used from target matrix 
    | % TODO: change getStanceTraj2 to only take 3x3 rotation matrix 
    | % Stance foot will rotate the body to desired orientation end of step 
    | endPoseRightTarget(1:3, 1:3) = Tb_fr1(1:3, 1:3); 
    | xyzqtrajr = getStanceTrajectory(endPoseRight, endPoseRightTarget, ...
    |                            measvec, Tw_fr0, STEPTIME, TS);
    | % xyzqtrajr = getStanceTraj2(endPoseRight, endPoseRightTarget, ...
    | %                            measvec, fholdx, fholdy);
    | 
    | 
    | end
  function calculateLeftTrajectories:
    | function calculateLeftTrajectories
    | Tb_bp = eye(4); % this is the change matrix, so reset everytime 
    | Tb_bp(1,1) =  cos(deltaYaw); Tb_bp(1,2) = sin(deltaYaw);
    | Tb_bp(2,1) = -sin(deltaYaw); Tb_bp(2,2) = cos(deltaYaw);
    | Tb_bp(1,4) = deltaPos(1);
    | Tb_bp(2,4) = deltaPos(2);
    | 
    | Tw_fl0 = Tw_b * TB_FL; % currrent world to right foot transform 
    | Tw_b = Tw_b * Tb_bp; 
    | Tw_fl1 = Tw_b * TB_FL; % next world to right foot transform 
    | Tw_fr = Tw_b * TB_FR;
    | % Tb_fr = Tb_bp * TB_FR; 
    | Tb_fl = Tb_bp * TB_FL; 
    | cxeos = Tw_fr(1,4);
    | cyeos = Tw_fr(2,4);
    | 
    | [cx, cy] = getCapturePoint(state0,W);
    | [px, py] = findZmp(cx, cy, W, STEPTIME, cxeos, cyeos);
    | u0 = [px py]';
    | fholdx = cx;
    | fholdy = cy;
    | Tw_fl1(1,4) = fholdx; Tw_fl1(2,4) = fholdy; 
    | 
    | idxmax = round(STEPTIME/TS);
    | [measvec, state1] = simulateLipm(state0, u0, idxmax);
    | state0 = state1;
    | % get world to new body pose based on state
    | Tw_bp = Tw_b;
    | Tw_bp(1,4) = state1(1); Tw_bp(2,4) = state1(3); 
    | % Get inverse
    | Tbp_w = eye(4);
    | Tbp_w(1:3,1:3) = Tw_bp(1:3,1:3)'; 
    | Tbp_w(1:3,4) = -Tw_bp(1:3,1:3)'*Tw_bp(1:3,4); 
    | Tbp_fr = Tbp_w * Tw_fr; 
    | 
    | endPoseRightTarget(1:3,1:3) = TB_FR(1:3,1:3);
    | Tw_b(1,4) = state1(1); Tw_b(2,4) = state1(3); 
    | Tb_w = TransformInverse(Tw_b); 
    | Tb_fr = Tb_w * Tw_fr; 
    | endPoseRightTarget(1,4) = Tb_fr(1,4);% cxeos - state1(1);
    | endPoseRightTarget(2,4) = Tb_fr(2,4);% cyeos - state1(3);
    | 
    | % tformtrajr = generateSwingTraj2(endPoseRight, endPoseRightTarget);
    | xyzqtrajr = generateSwingTraj(endPoseRight, endPoseRightTarget);
    | % stancetraj = getStanceTraj(measvec,fholdx,fholdy);
    | 
    | % only orientation will be used from target matrix 
    | endPoseLeftTarget(1:3, 1:3) = Tb_fl(1:3,1:3); 
    | xyzqtrajl = getStanceTrajectory(endPoseLeft, endPoseLeftTarget, ...
    |                            measvec, Tw_fl0, STEPTIME, TS); 
    | % xyzqtrajl = getStanceTraj2(endPoseLeft, endPoseLeftTarget, ...
    | %                            measvec, fholdx, fholdy);
    | end
  function xyzqtrajectory = getStanceTraj2(currMat,targetMat,liptraj,cpointx,cpointy):
    | function xyzqtrajectory = getStanceTraj2(currMat,targetMat,liptraj,cpointx,cpointy)
    | % 1) rotation
    | quat = quaternion(currMat(1:3,1:3), 'rotmat', 'frame'); 
    | quat = quat.compact; 
    | quattarget = quaternion(targetMat(1:3,1:3), 'rotmat', 'frame');
    | quattarget = quattarget.compact; 
    | 
    | pts0 = [0 0 0 quat]';
    | pts1 = [0 0 0 quattarget]'; 
    | 
    | wpts = [pts0 pts1]; 
    | tpts = [0 STEPTIME];
    | tvec = 0:TS:STEPTIME; 
    | 
    | [xyzqtrajectory, ~, ~, ~] = cubicpolytraj(wpts, tpts, tvec); 
    | 
    | % 2) position 
    | % transform body trajectory (w.r.t. world) to 
    | % foot trajectory (w.r.t. body) 
    | straj = -liptraj;
    | straj(1,:) = straj(1,:) + cpointx; 
    | straj(2,:) = straj(2,:) + cpointy; 
    | straj(3,:) = -ZMODEL; 
    | 
    | temp = length(xyzqtrajectory); 
    | xyzqtrajectory(1:3,1:temp) = straj(1:3,1:temp); 
    | end
  function tformtrajectory = generateSwingTraj2(currMat, targetMat):
    | function tformtrajectory = generateSwingTraj2(currMat, targetMat)
    | 
    | tpts = [0 STEPTIME];
    | tvec = 0:TS:STEPTIME; 
    | 
    | [tformtrajectory, ~, ~] = transformtraj(currMat,targetMat,tpts,tvec); 
    | end
  function xyzqtrajectory = getStanceTraj3(currMat,targetMat,Tw_b_traj,Tw_f_mat):
    | function xyzqtrajectory = getStanceTraj3(currMat,targetMat,Tw_b_traj,Tw_f_mat)
    | % 1) rotation
    | quat = quaternion(currMat(1:3,1:3), 'rotmat', 'frame'); 
    | quat = quat.compact; 
    | quattarget = quaternion(targetMat(1:3,1:3), 'rotmat', 'frame');
    | quattarget = quattarget.compact; 
    | 
    | pts0 = [0 0 0 quat]';
    | pts1 = [0 0 0 quattarget]'; 
    | 
    | wpts = [pts0 pts1]; 
    | tpts = [0 STEPTIME];
    | tvec = 0:TS:STEPTIME; 
    | 
    | [xyzqtrajectory, ~, ~, ~] = cubicpolytraj(wpts, tpts, tvec); 
    | 
    | % 2) position 
    | % transform body trajectory (w.r.t. world) to 
    | % foot trajectory (w.r.t. body) 
    | % footMat: world to foot at the beginning of step 
    | % liptraj: world to body 
    | % straj:   body to foot through the step
    | npoints = length(Tw_b_traj); 
    | Tliptraj = zeros(4,4,npoints); 
    | for idx2 = 1:npoints
    |     Tliptraj(4,4,idx2) = 1;
    |     % Get the rotational part of matrix from quaternion
    |     quat = quaternion(xyzqtrajectory(4:7,idx2)'); 
    |     Tliptraj(1:3,1:3,idx2) = quat.rotmat('frame');
    |     % Get the positional part from trajectory w.r.t. world  
    |     Tliptraj(1:3,4,idx2) = Tw_b_traj(1:3,idx2); 
    | end 
    | 
    | straj = zeros(3,npoints); 
    | for idx2 = 1:npoints
    |     temp1 = TransformInverse(Tliptraj(:,:,idx2)) * Tw_f_mat;
    |     straj(:,idx2) = temp1(1:3,4); 
    | end 
    | 
    | temp = length(xyzqtrajectory); 
    | xyzqtrajectory(1:3,1:temp) = straj(1:3,1:temp); 
    | end
